simulink model "no_friction"  (R2015a)
settings: Solver=ode45  StartTime=0.0  StopTime=10.0  FixedStep=0.0001  RelTol=1e-3
undefined symbols (not defined in the file): J, K, Ki, Kp, R, ref
settings Model: Creator=Max  LastModifiedBy=Max

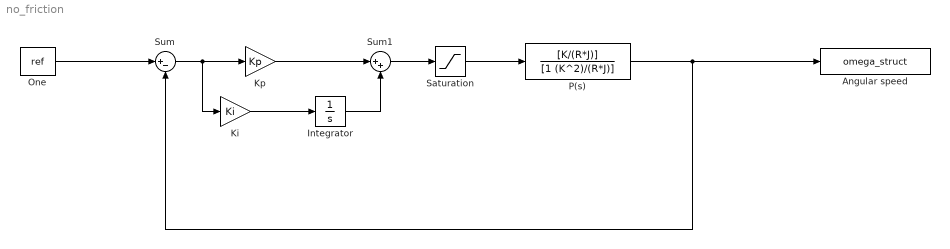
== system no_friction ==
  Angular speed : ToWorkspace  VariableName=omega_struct  SaveFormat=Structure With Time  SampleTime=-1
  Integrator : Integrator
  Ki : Gain  Gain=Ki
  Kp : Gain  Gain=Kp
  One : Constant  Value=ref
  P(s) : TransferFcn  Numerator=[K/(R*J)]  Denominator=[1 (K^2)/(R*J)]
  Saturation : Saturate  UpperLimit=6  LowerLimit=0
  Sum : Sum  Inputs=|+-
  Sum1 : Sum  Inputs=|++
  wires:
  One/1 -> Sum/1
  Sum/1 -> Ki/1, Kp/1
  Ki/1 -> Integrator/1
  Integrator/1 -> Sum1/2
  Kp/1 -> Sum1/1
  Sum1/1 -> Saturation/1
  Saturation/1 -> P(s)/1
  P(s)/1 -> Sum/2, Angular speed/1
